simulink model "dpd_fw_path_model"  (Simulink 8.7)
settings: Solver=VariableStepDiscrete  StartTime=0.0  StopTime=demo_dpd_param.endTime  RelTol=1e-3
PreLoadFcn:
  | % Run the setup script when the model is opened
  | setup_dpd_fw_path_model;
InitFcn:
  | % Run the setup script again just before the
  | % model is run, so that any updates made
  | % after opening are applied.
  | setup_dpd_fw_path_model;
undefined symbols (not defined in the file or in its folder): value
libraries: DSPBABase x7, DSPBAPrim x4, DSPBAUtilities x1, dpd_lib x1
Description:
  | DSP Builder Advanced Template for Template Design implementing Primitive Subsystems
settings Model: Creator=mjervis  LastModifiedBy=5g
settings DataIOCC: SignalLoggingSaveFormat=ModelDataLogs
settings OptimizationCC: ExpressionDepthLimit=2147483647
settings DebuggingCC: SolverPrmCheckMsg=warning  InheritedTsInSrcMsg=none  IntegerOverflowMsg=none  FcnCallInpInsideContextMsg=UseLocalSettings  AllowSymbolicDim=off  StateNameClashWarn=warning  IntegerSaturationMsg=none
settings GRTTargetCC: CombineOutputUpdateFcns=off  GRTInterface=on

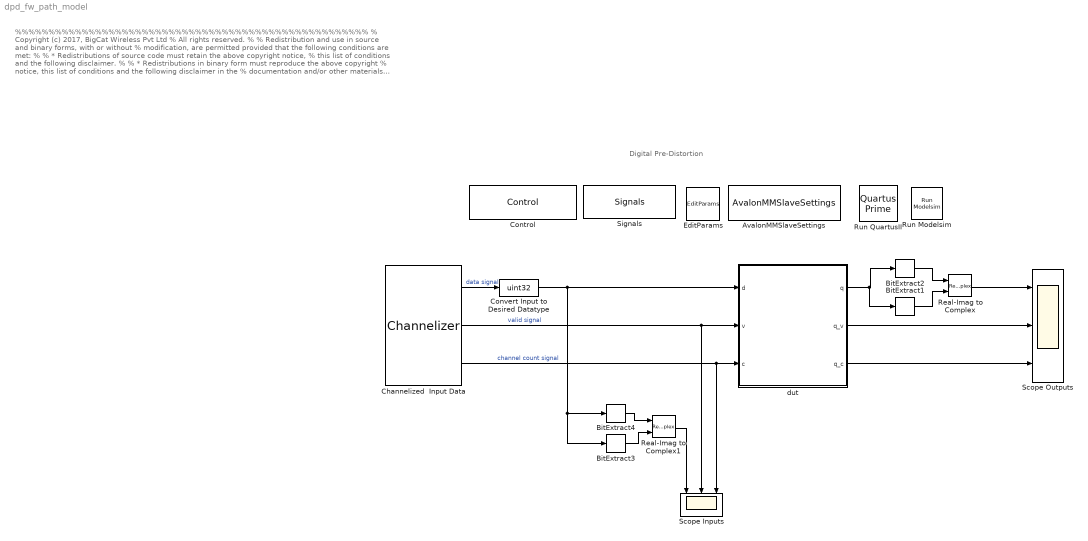
== system dpd_fw_path_model ==
  note: %%%%%%%%%%%%%%%%%%%%%%%%%%%%%%%%%%%%%%%%%%%%%%%%%%%%%
      |  % Copyright (c) 2017, BigCat Wireless Pvt Ltd
      |  % All rights reserved.
      |  %
      |  % Redistribution and use in source and binary forms, with or without
      |  % modification, are permitted provided that the following conditions are met:
      |  %
      |  %     * Redistributions of source code must retain the above copyright notice,
      |  %       this list of conditions and the following disclaimer.
      |  %
      |  %     * Redistributions in binary form must reproduce the above copyright
      |  %       notice, this list of conditions and the following disclaimer in the
      |  %       documentation and/or other materials provided with the distribution.
      |  %
      |  %     * Neither the name of the copyright holder nor the names of its contributors
      |  %       may be used to endorse or promote products derived from this software
      |  %       without specific prior written permission.
      |  %
      |  %
      |  %
      |  % THIS SOFTWARE IS PROVIDED BY THE COPYRIGHT HOLDERS AND CONTRIBUTORS "AS IS"
      |  % AND ANY EXPRESS OR IMPLIED WARRANTIES, INCLUDING, BUT NOT LIMITED TO, THE
      |  % IMPLIED WARRANTIES OF MERCHANTABILITY AND FITNESS FOR A PARTICULAR PURPOSE ARE
      |  % DISCLAIMED. IN NO EVENT SHALL THE COPYRIGHT HOLDER OR CONTRIBUTORS BE LIABLE
      |  % FOR ANY DIRECT, INDIRECT, INCIDENTAL, SPECIAL, EXEMPLARY, OR CONSEQUENTIAL
      |  % DAMAGES (INCLUDING, BUT NOT LIMITED TO, PROCUREMENT OF SUBSTITUTE GOODS OR
      |  % SERVICES; LOSS OF USE, DATA, OR PROFITS; OR BUSINESS INTERRUPTION) HOWEVER
      |  % CAUSED AND ON ANY THEORY OF LIABILITY, WHETHER IN CONTRACT, STRICT LIABILITY,
      |  % OR TORT (INCLUDING NEGLIGENCE OR OTHERWISE) ARISING IN ANY WAY OUT OF THE USE
      |  % OF THIS SOFTWARE, EVEN IF ADVISED OF THE POSSIBILITY OF SUCH DAMAGE.
      |  %
      |   %%%%%%%%%%%%%%%%%%%%%%%%%%%%%%%%%%%%%%%%%%%%%%%%%%%%%
  note: Digital Pre-Distortion
  AvalonMMSlaveSettings : DSPBABase/AvalonMMSlaveSettings
  BitExtract1 : DSPBAPrim/BitExtract  primtype=bitextract  nInputs=1  nOutputs=1  omode=Specify via dialog  otype=sfix(16)  scale=2^-15  rndmethod=Unbiased  factor=1  satmethod=Symmetric  shift_vec=[0 1 2 -1]  value=16  inPortNames=[' '; ' ';]  outPortNames=[' ']  dspbaimage=dspba_prim.jpg  text=fprintf('..%d', value);  style=Optimised  visibilities=8+1024  version=20090407
  BitExtract2 : DSPBAPrim/BitExtract  primtype=bitextract  nInputs=1  nOutputs=1  omode=Specify via dialog  otype=sfix(16)  scale=2^-15  rndmethod=Unbiased  factor=1  satmethod=Symmetric  shift_vec=[0 1 2 -1]  value=0  inPortNames=[' '; ' ';]  outPortNames=[' ']  dspbaimage=dspba_prim.jpg  text=fprintf('..%d', value);  style=Optimised  visibilities=8+1024  version=20090407
  BitExtract3 : DSPBAPrim/BitExtract  primtype=bitextract  nInputs=1  nOutputs=1  omode=Specify via dialog  otype=sfix(16)  scale=2^-15  rndmethod=Unbiased  factor=1  satmethod=Symmetric  shift_vec=[0 1 2 -1]  value=16  inPortNames=[' '; ' ';]  outPortNames=[' ']  dspbaimage=dspba_prim.jpg  text=fprintf('..%d', value);  style=Optimised  visibilities=8+1024  version=20090407
  BitExtract4 : DSPBAPrim/BitExtract  primtype=bitextract  nInputs=1  nOutputs=1  omode=Specify via dialog  otype=sfix(16)  scale=2^-15  rndmethod=Unbiased  factor=1  satmethod=Symmetric  shift_vec=[0 1 2 -1]  value=0  inPortNames=[' '; ' ';]  outPortNames=[' ']  dspbaimage=dspba_prim.jpg  text=fprintf('..%d', value);  style=Optimised  visibilities=8+1024  version=20090407
  Channelized  Input Data : DSPBAUtilities/Channelizer  data_input=demo_dpd_param.inputdata  folding=demo_dpd_param.Period  samples_valid=1  samples_idle=0  sample_time=1
  Control : DSPBABase/Control  generate=on  language=VHDL  destination=./rtl  destination_gui=./rtl  make_full_path=off  path_is_relative=on  autotestbench=on  signaldepth=2  coveragetestbench=off  logs=off  spacewidth=2  spacenum=1  addrwidth=10  datawidth=32  dataendian=Big Endian  hierarchicalnames=off  ramThresholdBits=-1  distRamThresholdBits=-1  mlabThresholdBits=-1  hardMultiplierThresholdLuts=-1  version=20090407  errorOnChanMismatch=1  errorOnGPIOMismatch=0  importModelsimResults=0  cycleAccurate=off  reinterpretCastMult=off  paramFile=dpd_fw_path_model_params.xml
  Convert Input to Desired Datatype : DataTypeConversion  OutDataTypeStr=uint32  RndMeth=Convergent  SaturateOnIntegerOverflow=on
  EditParams : DSPBABase/EditParams  version=20090407
  Real-Imag to Complex : RealImagToComplex
  Real-Imag to Complex1 : RealImagToComplex
  Run Modelsim : DSPBABase/Run Modelsim  version=20090407
  "Run QuartusII " : DSPBABase/Quartus Prime  version=20090407
  Scope Inputs : Scope  NumInputPorts=3
  Scope Outputs : Scope  NumInputPorts=3
  Signals : DSPBABase/Signals  clk=clk  freq=demo_dpd_param.ClockRate  margin=demo_dpd_param.ClockMargin  rst=areset  rstactive=High  bus=bus  enbusclock=off  busfreq=245.76  bussync=off  version=20090407
  dut : Subsystem
  wires:
  Channelized  Input Data/1 -> Convert Input to Desired Datatype/1  "data signal"
  Channelized  Input Data/2 -> Scope Inputs/2, dut/2(v)  "valid signal"
  Channelized  Input Data/3 -> Scope Inputs/3, dut/3(c)  "channel count signal"
  dut/2(q_v) -> Scope Outputs/2
  dut/3(q_c) -> Scope Outputs/3
  BitExtract1/1 -> Real-Imag to Complex/2
  BitExtract2/1 -> Real-Imag to Complex/1
  Real-Imag to Complex/1 -> Scope Outputs/1
  dut/1(q) -> BitExtract1/1, BitExtract2/1
  BitExtract3/1 -> Real-Imag to Complex1/2
  BitExtract4/1 -> Real-Imag to Complex1/1
  Real-Imag to Complex1/1 -> Scope Inputs/1
  Convert Input to Desired Datatype/1 -> BitExtract4/1, BitExtract3/1, dut/1(d)

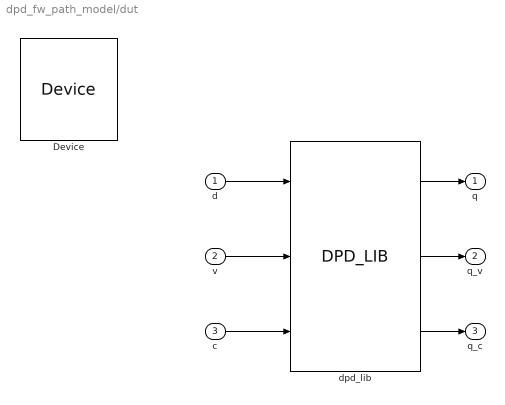
== system dpd_fw_path_model/dut ==
  d : Inport
  v : Inport  Port=2
  c : Inport  Port=3
  Device : DSPBABase/Device  family=Arria 10  deviceMember=Arria 10  stratix4device=Stratix IV E  hardcopy4device=HardCopy IV E  stratix5device=Stratix V GX  device=AUTO  speed=1  stratixSpeed=-5  stratix2Speed=-3  stratix3Speed=-2  stratix4gxSpeed=-2  stratix4gtSpeed=-1  cyclone2Speed=-6  cyclone3Speed=-7  arria2Speed=-4  cyclone4eSpeed=-8  stratix5Speed=-3  arria5Speed=-4  arriaSpeed=-6  cyclone3lsSpeed=-7  cyclone5Speed=-6  arria2gzSpeed=-3  nightFurySpeed=-2  ecp2Speed=-7  hardcopycompat=off  version=20140217  max10flashmode=off  max10nomeminit=off
  dpd_lib : dpd_lib/DPD_LIB  CoefWidth=Coeff_width  Coeff_fractionwidth=Coeff_fractionwidth  DataWidth=WordLength  fractionwidth=FractionLength  Lateny=Latency  ClockMargin=demo_dpd_param.ClockMargin  Pipeline_stages=pipeline_Stages  LutContent=LUTS.ENTRIES
      link override dpd/ChannelOut1: latency=49
  q : Outport
  q_v : Outport  Port=2
  q_c : Outport  Port=3
  wires:
  d/1 -> dpd_lib/1
  v/1 -> dpd_lib/2
  c/1 -> dpd_lib/3
  dpd_lib/2 -> q_v/1
  dpd_lib/3 -> q_c/1
  dpd_lib/1 -> q/1
